simulink model "untitled1"  (R2014a)
settings: Solver=ode45  StartTime=0.0  StopTime=10.0  RelTol=1e-3
settings Model: Creator=Algot  LastModifiedBy=Algot

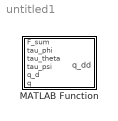
== system untitled1 ==
  MATLAB Function : MATLAB Function  TreatAsAtomicUnit=on

== matlab function untitled1/MATLAB Function ==
  data: F_sum input; q_dd output; tau_phi input; tau_theta input; tau_psi input; q_d input; q input
function q_dd = fcn(F_sum, tau_phi, tau_theta, tau_psi, q_d, q)
%#codegen

q_dd = F_sum;
